simulink model "FeatureExtractionApp"  (R2018a)
settings: Solver=FixedStepAuto  StartTime=0.0  StopTime=10.0  RelTol=1e-3
undefined symbols (not defined in the file or in its folder): Data_Display, ftrapp
libraries: androidsensorlib x2, androiduilib x1, androidcommunicationlib x1
settings Model: Creator=MUGDHO  LastModifiedBy=MUGDHO
settings OptimizationCC: EnhancedBackFolding=on  PassReuseOutputArgsAs=Individual arguments  MaxStackSize=64  OptimizeBlockOrder=speed  DifferentSizesBufferReuse=on  OptimizationCustomize=off
settings DebuggingCC: ParameterTunabilityLossMsg=error
settings HardwareCC: ProdBitPerPointer=32  ProdBitPerSizeT=32  ProdBitPerPtrDiffT=32  ProdLargestAtomicInteger=Long  ProdLargestAtomicFloat=Double  ProdWordSize=32  ProdHWDeviceType=ARM Compatible->ARM Cortex
settings SFSimCC: MATLABDynamicMemAlloc=off
settings RTWCC: SystemTargetFile=ert.tlc  HardwareBoard=Android Device  TLCOptions="-aInlineSetEventsForThisBaseRateFcn=TLC_FALSE -aSuppressMultiTaskScheduler=TLC_FALSE  -aRateBasedStepFcn=0"  TemplateMakefile=ert_default_tmf  GenerateReport=on  RTWVerbose=off  Toolchain=Android SDK/NDK Tools  IncludeHyperlinkInReport=on  LaunchReport=on  GenerateTraceInfo=on  GenerateTraceReport=on  GenerateTraceReportSl=on  GenerateTraceReportSf=on  GenerateTraceReportEml=on
settings CodeAppCC: ForceParamTrailComments=on  IgnoreCustomStorageClasses=off  OperatorAnnotations=on  SimulinkDataObjDesc=on  SFDataObjDesc=on  InsertBlockDesc=on

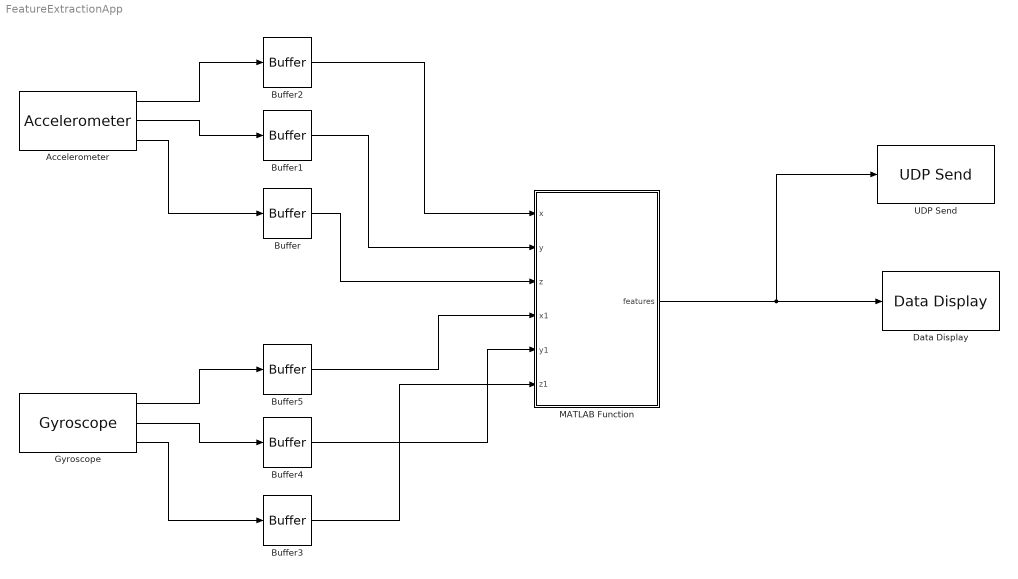
== system FeatureExtractionApp ==
  Accelerometer : androidsensorlib/Accelerometer  OutputVector=off  SampleTime=.01  BlockPlatform=Android
      settings: SourceProductName=Simulink Support Package for Android Devices  SourceProductBaseCode=ANDROID
  Buffer{,1..5} (6 alike) : Buffer  N=150  OutputFrames=off
  Data Display : androiduilib/Data Display  DataDisplayId=ftrapp/Data_Display  Format=Float  Precision=6  SimulateUsing=Code generation  blockPlatform=Android
      settings: SourceProductName=Simulink Support Package for Android Devices  SourceProductBaseCode=ANDROID
  Gyroscope : androidsensorlib/Gyroscope  OutputVector=off  SampleTime=.01  BlockPlatform=Android
      settings: SourceProductName=Simulink Support Package for Android Devices  SourceProductBaseCode=ANDROID
  MATLAB Function : MATLAB Function  TreatAsAtomicUnit=on
  UDP Send : androidcommunicationlib/UDP Send  remoteURL='255.255.255.255'  remotePort=25005  localURL='0.0.0.0'  localPortSource=Automatically determine  localPort=-1  sampletime=-1  blockPlatform=Android  separateLengthPort=0
      settings: SourceProductName=Simulink Support Package for Android Devices  SourceProductBaseCode=ANDROID
  wires:
  Accelerometer/1 -> Buffer2/1
  Accelerometer/2 -> Buffer1/1
  Accelerometer/3 -> Buffer/1
  Gyroscope/3 -> Buffer3/1
  Gyroscope/1 -> Buffer5/1
  Gyroscope/2 -> Buffer4/1
  Buffer2/1 -> MATLAB Function/1(x)
  Buffer1/1 -> MATLAB Function/2(y)
  Buffer/1 -> MATLAB Function/3(z)
  Buffer5/1 -> MATLAB Function/4(x1)
  Buffer4/1 -> MATLAB Function/5(y1)
  Buffer3/1 -> MATLAB Function/6(z1)
  MATLAB Function/1(features) -> UDP Send/1, Data Display/1

== matlab function FeatureExtractionApp/MATLAB Function ==
  data: x input; features output; y input; z input; x1 input; y1 input; z1 input
function features = ftrextrct(x,y,z,x1,y1,z1)
 
 n = length(x);
 frs = n;
 a0 = [x y z]';
 g0 = [x1 y1 z1]';
 b = (sum(a0'))'/n;
 q1 = atan(b(2)/b(3));
 q2 = atan(b(1)/(b(2)*sin(q1)+b(3)*cos(q1)));
 r1 = [cos(q2) -sin(q1)*sin(q2) -cos(q1)*sin(q2)];
 r2 = [0 cos(q1) -sin(q1)];
 r3 = [sin(q2) sin(q1)*cos(q2) cos(q1)*cos(q2)];
 r = [r1;r2;r3];
 a1 = r*a0;
 g1 = r*g0;
 a1z = sum(a1(3,:))/n;
 a2 = [a1(1,:);a1(2,:);a1(3,:)-a1z];
 ah = sqrt(a2(1,:).^2 + a2(2,:).^2);
 av = abs(a2(3,:));
 gh = sqrt(g1(1,:).^2 + g1(2,:).^2);
 gv = abs(g1(3,:));
 eah = sum(ah.^2)/frs;
 eav = sum(av.^2)/frs;
 egh = sum(gh.^2)/frs;
 egv = sum(gv.^2)/frs;
 rms = [eav eah egv egh];
 actv = var(av);
 acth = var(ah);
 activity = [actv acth];
 mobv = std(diff(av))./std(av);
 mobh = std(diff(ah))./std(ah);
 mobility = [mobv mobh];
 compv = std(diff(diff(av)))./std(diff(av))./mobv;
 comph = std(diff(diff(ah)))./std(diff(ah))./mobh;
 complexity = [compv comph];
 maxa = [max(a2(1,:)) max(a2(2,:)) max(a2(3,:))];
 maxg = [max(g1(1,:)) max(g1(2,:)) max(g1(3,:))];
 maxval = [maxa maxg];
 maxca = [max(xcorr(a2(1,:))) max(xcorr(a2(2,:))) max(xcorr(a2(3,:)))];
 maxcg = [max(xcorr(g1(1,:))) max(xcorr(g1(2,:))) max(xcorr(g1(3,:)))];
 maxcorr = [maxca maxcg];
 meana = [mean(abs(a2(1,:))) mean(abs(a2(2,:))) mean(abs(a2(3,:)))];
 meang = [mean(abs(g1(1,:))) mean(abs(g1(2,:))) mean(abs(g1(3,:)))];
 meanval = [meana meang];
 feature = [meanval rms maxval maxcorr activity mobility complexity];
 features = feature;
